simulink library "CommonMetricsBlock"  (R2018b)
settings: Solver=VariableStepAuto  StartTime=0.0  StopTime=10.0  RelTol=1e-3
libraries: simulink x4, CalcMinDist x3
settings Model: Creator=BI28030  LastModifiedBy=BI28030

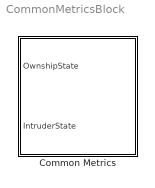
== system CommonMetricsBlock ==
  Common Metrics : Subsystem  mask(CommonMetrics){}
      mask help:
      | Calculates metrics common to all aircraft encounters, those having to do with the separation
      | between aircraft. Metrics pertaining to the operation of advisory systems (e.g. alert rate) are not
      | included in this block.
      |
      | The calculated metrics are saved to a workspace.
      mask Help:
      | Calculates metrics common to all aircraft encounters, those having to do with the separation
      | between aircraft. Metrics pertaining to the operation of advisory systems (e.g. alert rate) are not
      | included in this block.
      | 
      | The calculated metrics are saved to a workspace.
      | 
      | INPUTS
      | ==========
      | Aircraft1 - A CASSATT v6 AircraftState bus from first aircraft
      | Aircraft2 - A CASSATT v6 AircraftState bus from second aircraft
      | 
      | OUTPUTS (Saved to Workspace)
      | ==========
      | NMAC - Near Mid Air Collision.  True if the separation between the two
      |     aircraft has ever been simultaneously less than 100 feet vertically and
      |     500 feet horizontally.
      | hmd_ft - Horizontal Miss Distance in feet.  The minimum horizontal
      |     separation that has occurred between the two aircraft.
      | vmd_ft - Vertical Miss Distance in feet.  The vertical separation of the
      |     two aircaft at the Time of Closest Approach.
      | tca - Time of Closest Approach in seconds.  Prior to horizontal separation
      |     of less than 500 feet, the Time of Closest Approach is the time when
      |     the minimum horizontal separation was achieved.  Once horizontal
      |     separation has been less than 500 feet, the Time of Closest Approach is
      |     when minimum vertical separation occurs while horizontal separation is
      |     less than 500 feet.

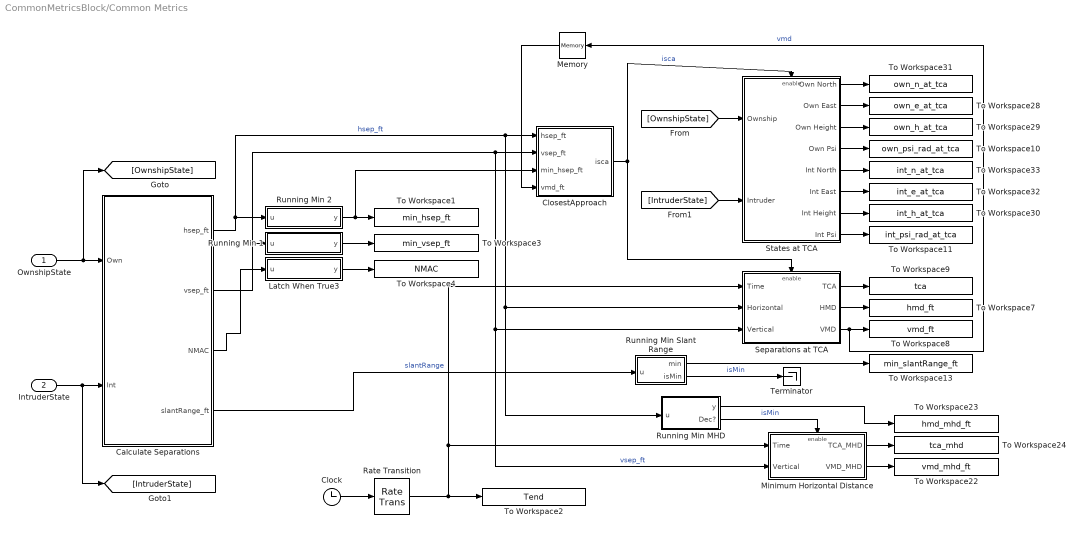
== system CommonMetricsBlock/Common Metrics ==
  OwnshipState : Inport  OutDataTypeStr=Bus: AircraftState  PortDimensions=1
  IntruderState : Inport  Port=2  OutDataTypeStr=Bus: AircraftState  PortDimensions=1
  Calculate Separations : Subsystem
  Clock : Clock
  ClosestApproach : Subsystem
  Latch When True3 : Subsystem
      mask Display: disp('Latch when true')
  Memory : Memory
  Minimum Horizontal Distance : Subsystem  TreatAsAtomicUnit=on
  Rate Transition : RateTransition
  Running Min 1 : Subsystem
      mask Display: disp('Running min')
  Running Min 2 : Subsystem
      mask Display: disp('Running min')
  Running Min MHD : Subsystem
  Running Min Slant Range : Subsystem
  Separations at TCA : Subsystem  TreatAsAtomicUnit=on
  States at TCA : Subsystem  TreatAsAtomicUnit=on
  Terminator : Terminator
  To Workspace1 : ToWorkspace  VariableName=min_hsep_ft  SampleTime=-1
      settings: MaxDataPoints=1
  To Workspace10 : ToWorkspace  VariableName=own_psi_rad_at_tca  SampleTime=-1
      settings: MaxDataPoints=1
  To Workspace11 : ToWorkspace  VariableName=int_psi_rad_at_tca  SampleTime=-1
      settings: MaxDataPoints=1
  To Workspace13 : ToWorkspace  VariableName=min_slantRange_ft  SampleTime=-1
      settings: MaxDataPoints=1
  To Workspace2 : ToWorkspace  VariableName=Tend  SampleTime=-1
      settings: MaxDataPoints=1
  To Workspace22 : ToWorkspace  VariableName=vmd_mhd_ft  SampleTime=-1
      settings: MaxDataPoints=1
  To Workspace23 : ToWorkspace  VariableName=hmd_mhd_ft  SampleTime=-1
      settings: MaxDataPoints=1
  To Workspace24 : ToWorkspace  VariableName=tca_mhd  SampleTime=-1
      settings: MaxDataPoints=1
  To Workspace28 : ToWorkspace  VariableName=own_e_at_tca  SampleTime=-1
      settings: MaxDataPoints=1
  To Workspace29 : ToWorkspace  VariableName=own_h_at_tca  SampleTime=-1
      settings: MaxDataPoints=1
  To Workspace3 : ToWorkspace  VariableName=min_vsep_ft  SampleTime=-1
      settings: MaxDataPoints=1
  To Workspace30 : ToWorkspace  VariableName=int_h_at_tca  SampleTime=-1
      settings: MaxDataPoints=1
  To Workspace31 : ToWorkspace  VariableName=own_n_at_tca  SampleTime=-1
      settings: MaxDataPoints=1
  To Workspace32 : ToWorkspace  VariableName=int_e_at_tca  SampleTime=-1
      settings: MaxDataPoints=1
  To Workspace33 : ToWorkspace  VariableName=int_n_at_tca  SampleTime=-1
      settings: MaxDataPoints=1
  To Workspace4 : ToWorkspace  VariableName=NMAC  SampleTime=-1
      settings: MaxDataPoints=1
  To Workspace7 : ToWorkspace  VariableName=hmd_ft  SampleTime=-1
      settings: MaxDataPoints=1
  To Workspace8 : ToWorkspace  VariableName=vmd_ft  SampleTime=-1
      settings: MaxDataPoints=1
  To Workspace9 : ToWorkspace  VariableName=tca  SampleTime=-1
      settings: MaxDataPoints=1
  wires:
  States at TCA/8(Int Psi) -> To Workspace11/1
  States at TCA/4(Own Psi) -> To Workspace10/1
  Memory/1 -> ClosestApproach/4(vmd_ft)
  OwnshipState/1 -> [OwnshipState], Calculate Separations/1(Own)
  [IntruderState] -> States at TCA/2(Intruder)
  [OwnshipState] -> States at TCA/1(Ownship)
  States at TCA/7(Int Height) -> To Workspace30/1
  States at TCA/6(Int East) -> To Workspace32/1
  States at TCA/5(Int North) -> To Workspace33/1
  States at TCA/3(Own Height) -> To Workspace29/1
  States at TCA/2(Own East) -> To Workspace28/1
  States at TCA/1(Own North) -> To Workspace31/1
  ClosestApproach/1(isca) -> States at TCA/Enable, Separations at TCA/Enable  "isca"
  Calculate Separations/1(hsep_ft) -> Running Min MHD/1(u), Separations at TCA/2(Horizontal), ClosestApproach/1(hsep_ft), Running Min 2/1(u)  "hsep_ft"
  Running Min Slant Range/1(min) -> To Workspace13/1
  Calculate Separations/4(slantRange_ft) -> Running Min Slant Range/1(u)  "slantRange"
  Running Min 1/1(y) -> To Workspace3/1
  Separations at TCA/2(HMD) -> To Workspace7/1
  Calculate Separations/3(NMAC) -> Latch When True3/1(u)
  IntruderState/1 -> [IntruderState], Calculate Separations/2(Int)
  Latch When True3/1(y) -> To Workspace4/1
  Separations at TCA/1(TCA) -> To Workspace9/1
  Clock/1 -> Rate Transition/1
  Separations at TCA/3(VMD) -> Memory/1, To Workspace8/1  "vmd"
  Running Min 2/1(y) -> ClosestApproach/3(min_hsep_ft), To Workspace1/1
  Running Min Slant Range/2(isMin) -> Terminator/1  "isMin"
  Running Min MHD/2(Dec?) -> Minimum Horizontal Distance/Enable  "isMin"
  Running Min MHD/1(y) -> To Workspace23/1
  Minimum Horizontal Distance/2(VMD_MHD) -> To Workspace22/1
  Minimum Horizontal Distance/1(TCA_MHD) -> To Workspace24/1
  Rate Transition/1 -> Minimum Horizontal Distance/1(Time), Separations at TCA/1(Time), To Workspace2/1
  Calculate Separations/2(vsep_ft) -> Running Min 1/1(u), Minimum Horizontal Distance/2(Vertical), Separations at TCA/3(Vertical), ClosestApproach/2(vsep_ft)  "vsep_ft"

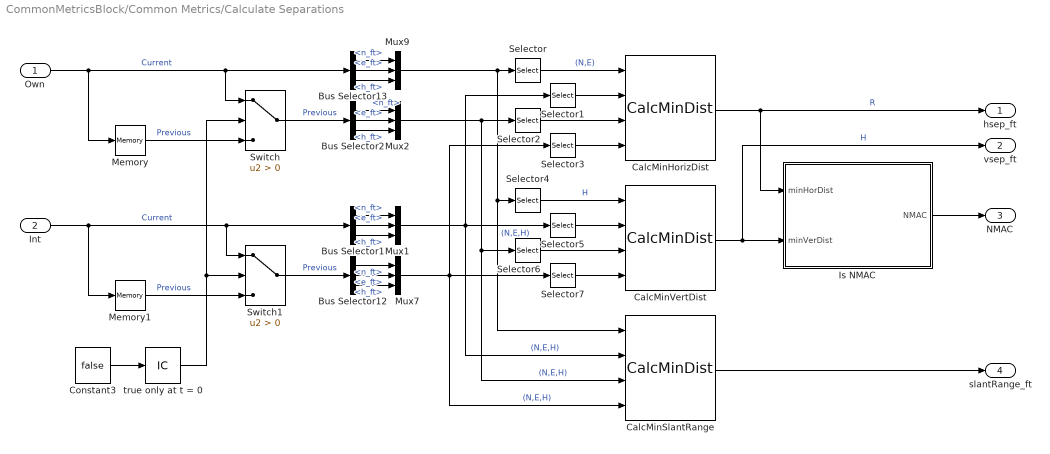
== system CommonMetricsBlock/Common Metrics/Calculate Separations ==
  Own : Inport
  Int : Inport  Port=2
  Bus Selector{1..2,12..13} (4 alike) : BusSelector  OutputSignals=n_ft,e_ft,h_ft
  CalcMinHorizDist : CalcMinDist/CalcMinDist
      settings: SourceProductName=CASSATTv6: Metrics Library
  CalcMinSlantRange : CalcMinDist/CalcMinDist
      settings: SourceProductName=CASSATTv6: Metrics Library
  CalcMinVertDist : CalcMinDist/CalcMinDist
      settings: SourceProductName=CASSATTv6: Metrics Library
  Constant3 : Constant  Value=false  SampleTime=Inf
  Is NMAC : Subsystem
  Memory : Memory
  Memory1 : Memory
  Mux{1..2,7,9} (4 alike) : Mux  Inputs=3
  Selector{,1..3} (4 alike) : Selector  InputPortWidth=3  IndexOptions=Index vector (dialog)  Indices=[1 2]  OutputSizes=1
  Selector{4..7} (4 alike) : Selector  InputPortWidth=3  IndexOptions=Index vector (dialog)  Indices=3  OutputSizes=1
  Switch : Switch  Criteria=u2 > Threshold
  Switch1 : Switch  Criteria=u2 > Threshold
  true only at t = 0 : InitialCondition  Value=true
  hsep_ft : Outport
  vsep_ft : Outport  Port=2
  NMAC : Outport  Port=3
  slantRange_ft : Outport  Port=4
  wires:
  Is NMAC/1(NMAC) -> NMAC/1
  Selector7/1 -> CalcMinVertDist/4
  Selector6/1 -> CalcMinVertDist/3
  Selector5/1 -> CalcMinVertDist/2
  Selector4/1 -> CalcMinVertDist/1  "H"
  Selector3/1 -> CalcMinHorizDist/4
  Selector2/1 -> CalcMinHorizDist/3
  Selector1/1 -> CalcMinHorizDist/2
  Selector/1 -> CalcMinHorizDist/1  "(N,E)"
  Mux2/1 -> Selector2/1, CalcMinSlantRange/3, Selector6/1  "(N,E,H)"
  Mux1/1 -> CalcMinSlantRange/2, Selector5/1, Selector1/1  "(N,E,H)"
  Bus Selector2/3 -> Mux2/3  "<h_ft>"
  Bus Selector2/2 -> Mux2/2  "<e_ft>"
  Bus Selector2/1 -> Mux2/1  "<n_ft>"
  Switch/1 -> Bus Selector2/1  "Previous"
  Bus Selector1/3 -> Mux1/3  "<h_ft>"
  Bus Selector1/2 -> Mux1/2  "<e_ft>"
  Bus Selector1/1 -> Mux1/1  "<n_ft>"
  Bus Selector13/3 -> Mux9/3  "<h_ft>"
  Bus Selector13/2 -> Mux9/2  "<e_ft>"
  Bus Selector13/1 -> Mux9/1  "<n_ft>"
  CalcMinVertDist/1 -> Is NMAC/2(minVerDist), vsep_ft/1  "H"
  Switch1/1 -> Bus Selector12/1  "Previous"
  Own/1 -> Switch/1, Bus Selector13/1, Memory/1  "Current"
  Int/1 -> Memory1/1, Switch1/1, Bus Selector1/1  "Current"
  CalcMinSlantRange/1 -> slantRange_ft/1
  Mux7/1 -> CalcMinSlantRange/4, Selector7/1, Selector3/1  "(N,E,H)"
  Bus Selector12/3 -> Mux7/3  "<h_ft>"
  Bus Selector12/1 -> Mux7/1  "<n_ft>"
  Bus Selector12/2 -> Mux7/2  "<e_ft>"
  Mux9/1 -> CalcMinSlantRange/1, Selector4/1, Selector/1  "(N,E,H)"
  Memory/1 -> Switch/3  "Previous"
  Memory1/1 -> Switch1/3  "Previous"
  Constant3/1 -> true only at t = 0/1
  true only at t = 0/1 -> Switch1/2, Switch/2
  CalcMinHorizDist/1 -> hsep_ft/1, Is NMAC/1(minHorDist)  "R"

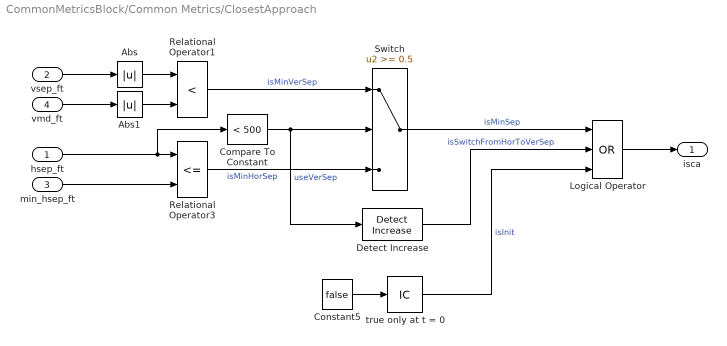
== system CommonMetricsBlock/Common Metrics/ClosestApproach ==
  hsep_ft : Inport
  vsep_ft : Inport  Port=2
  min_hsep_ft : Inport  Port=3
  vmd_ft : Inport  Port=4
  Abs : Abs
  Abs1 : Abs
  Compare To Constant : simulink/Logic and Bit Operations/Compare To Constant  relop=<  const=500  OutDataTypeStr=boolean
  Constant5 : Constant  Value=false  SampleTime=Inf
  Detect Increase : simulink/Logic and Bit Operations/Detect Increase  vinit=0.0  OutDataTypeStr=boolean
  Logical Operator : Logic  Operator=OR  Inputs=3  AllPortsSameDT=off  OutDataTypeStr=boolean
  Relational Operator1 : RelationalOperator  Operator=<  OutDataTypeStr=boolean  RndMeth=Nearest
  Relational Operator3 : RelationalOperator  Operator=<=  OutDataTypeStr=boolean  RndMeth=Nearest
  Switch : Switch  Threshold=0.5
  true only at t = 0 : InitialCondition  Value=true
  isca : Outport
  wires:
  true only at t = 0/1 -> Logical Operator/3  "isInit"
  Constant5/1 -> true only at t = 0/1
  Relational Operator3/1 -> Switch/3  "isMinHorSep"
  min_hsep_ft/1 -> Relational Operator3/2
  Relational Operator1/1 -> Switch/1  "isMinVerSep"
  Abs/1 -> Relational Operator1/1
  Abs1/1 -> Relational Operator1/2
  vmd_ft/1 -> Abs1/1
  vsep_ft/1 -> Abs/1
  Switch/1 -> Logical Operator/1  "isMinSep"
  Compare To Constant/1 -> Detect Increase/1, Switch/2  "useVerSep"
  hsep_ft/1 -> Relational Operator3/1, Compare To Constant/1
  Logical Operator/1 -> isca/1
  Detect Increase/1 -> Logical Operator/2  "isSwitchFromHorToVerSep"

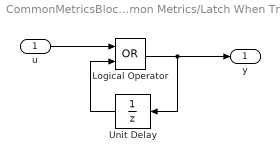
== system CommonMetricsBlock/Common Metrics/Latch When True3 ==
  u : Inport  PortDimensions=1
  Logical Operator : Logic  Operator=OR  AllPortsSameDT=off  OutDataTypeStr=boolean
  Unit Delay : UnitDelay  SampleTime=-1
  y : Outport
  wires:
  u/1 -> Logical Operator/1
  Logical Operator/1 -> y/1, Unit Delay/1
  Unit Delay/1 -> Logical Operator/2

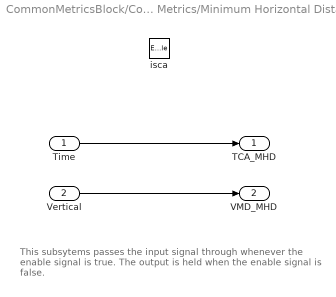
== system CommonMetricsBlock/Common Metrics/Minimum Horizontal Distance ==
  note: This subsytems passes the input signal through whenever the enable signal is true. The output is held when the enable signal is false.
  Time : Inport
  Vertical : Inport  Port=2
  isca : EnablePort
  TCA_MHD : Outport
  VMD_MHD : Outport  Port=2
  wires:
  Time/1 -> TCA_MHD/1
  Vertical/1 -> VMD_MHD/1

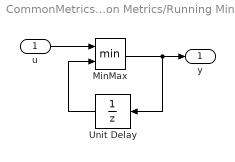
== system CommonMetricsBlock/Common Metrics/Running Min 1 ==
  u : Inport  PortDimensions=1
  MinMax : MinMax  Inputs=2
  Unit Delay : UnitDelay  InitialCondition=NaN  SampleTime=-1
  y : Outport
  wires:
  Unit Delay/1 -> MinMax/2
  MinMax/1 -> Unit Delay/1, y/1
  u/1 -> MinMax/1

== system CommonMetricsBlock/Common Metrics/Running Min 2 ==
  u : Inport  PortDimensions=1
  MinMax : MinMax  Inputs=2
  Unit Delay : UnitDelay  InitialCondition=NaN  SampleTime=-1
  y : Outport
  wires:
  u/1 -> MinMax/1
  MinMax/1 -> y/1, Unit Delay/1
  Unit Delay/1 -> MinMax/2

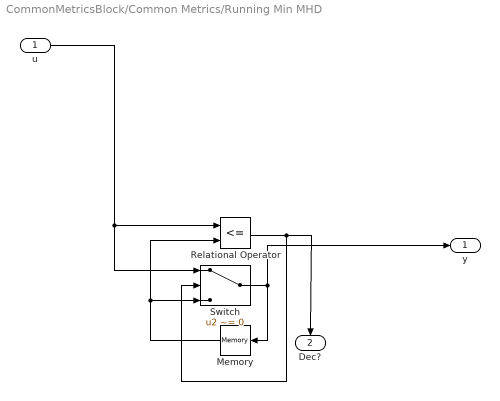
== system CommonMetricsBlock/Common Metrics/Running Min MHD ==
  u : Inport
  Memory : Memory  InitialCondition=42000000
  Relational Operator : RelationalOperator  Operator=<=  OutDataTypeStr=boolean  RndMeth=Nearest
  Switch : Switch  Criteria=u2 ~= 0
  y : Outport
  Dec? : Outport  Port=2
  wires:
  Switch/1 -> y/1, Memory/1
  Memory/1 -> Switch/3, Relational Operator/2
  u/1 -> Switch/1, Relational Operator/1
  Relational Operator/1 -> Dec?/1, Switch/2

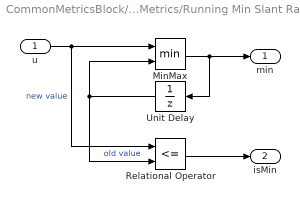
== system CommonMetricsBlock/Common Metrics/Running Min Slant Range ==
  u : Inport
  MinMax : MinMax  Inputs=2
  Relational Operator : RelationalOperator  Operator=<=  OutDataTypeStr=boolean  RndMeth=Nearest
  Unit Delay : UnitDelay  InitialCondition=inf  SampleTime=-1
  min : Outport
  isMin : Outport  Port=2
  wires:
  u/1 -> MinMax/1, Relational Operator/1  "new value"
  MinMax/1 -> min/1, Unit Delay/1
  Unit Delay/1 -> Relational Operator/2, MinMax/2  "old value"
  Relational Operator/1 -> isMin/1

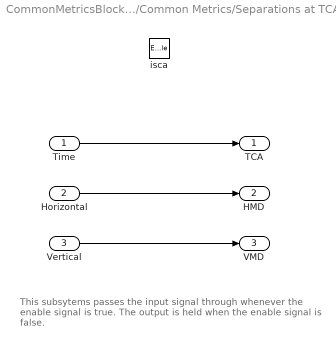
== system CommonMetricsBlock/Common Metrics/Separations at TCA ==
  note: This subsytems passes the input signal through whenever the enable signal is true. The output is held when the enable signal is false.
  Time : Inport
  Horizontal : Inport  Port=2
  Vertical : Inport  Port=3
  isca : EnablePort
  TCA : Outport
  HMD : Outport  Port=2
  VMD : Outport  Port=3
  wires:
  Vertical/1 -> VMD/1
  Horizontal/1 -> HMD/1
  Time/1 -> TCA/1

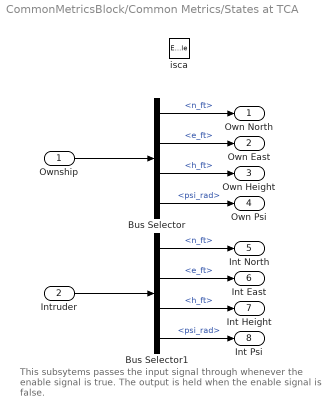
== system CommonMetricsBlock/Common Metrics/States at TCA ==
  note: This subsytems passes the input signal through whenever the enable signal is true. The output is held when the enable signal is false.
  Ownship : Inport
  Intruder : Inport  Port=2
  isca : EnablePort
  Bus Selector : BusSelector  OutputSignals=n_ft,e_ft,h_ft,psi_rad
  Bus Selector1 : BusSelector  OutputSignals=n_ft,e_ft,h_ft,psi_rad
  Own North : Outport
  Own East : Outport  Port=2
  Own Height : Outport  Port=3
  Own Psi : Outport  Port=4
  Int North : Outport  Port=5
  Int East : Outport  Port=6
  Int Height : Outport  Port=7
  Int Psi : Outport  Port=8
  wires:
  Bus Selector1/4 -> Int Psi/1  "<psi_rad>"
  Bus Selector/4 -> Own Psi/1  "<psi_rad>"
  Bus Selector1/3 -> Int Height/1  "<h_ft>"
  Bus Selector1/2 -> Int East/1  "<e_ft>"
  Bus Selector1/1 -> Int North/1  "<n_ft>"
  Bus Selector/3 -> Own Height/1  "<h_ft>"
  Bus Selector/2 -> Own East/1  "<e_ft>"
  Bus Selector/1 -> Own North/1  "<n_ft>"
  Intruder/1 -> Bus Selector1/1
  Ownship/1 -> Bus Selector/1

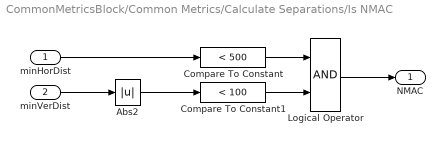
== system CommonMetricsBlock/Common Metrics/Calculate Separations/Is NMAC ==
  minHorDist : Inport
  minVerDist : Inport  Port=2
  Abs2 : Abs
  Compare To Constant : simulink/Logic and Bit Operations/Compare To Constant  relop=<  const=500  OutDataTypeStr=boolean
  Compare To Constant1 : simulink/Logic and Bit Operations/Compare To Constant  relop=<  const=100  OutDataTypeStr=boolean
  Logical Operator : Logic  AllPortsSameDT=off  OutDataTypeStr=boolean
  NMAC : Outport
  wires:
  Abs2/1 -> Compare To Constant1/1
  Compare To Constant1/1 -> Logical Operator/2
  Logical Operator/1 -> NMAC/1
  Compare To Constant/1 -> Logical Operator/1
  minVerDist/1 -> Abs2/1
  minHorDist/1 -> Compare To Constant/1
